simulink model "acvh_controller_mark0"  (R2020b)
settings: Solver=FixedStepAuto  StartTime=0.0  StopTime=Inf  RelTol=1e-3
values from neighbouring files (symbols this model uses):
  SampleTime = 0.001    [iris_quadcopter_specs.m]
undefined symbols (not defined in the file or in its folder): dev, Main, pwm_output0
libraries: pid_lib x6, px4uORBlib x5, sharedtransform x1, px4lib x1
settings Model: SimulationMode=external  EnablePacing=on  PacingRate=0.008900  ExtModeTrigDuration=10  Creator=sid  LastModifiedBy=sid
settings SolverCC: PositivePriorityOrder=on  AutoInsertRateTranBlk=on
settings OptimizationCC: EnhancedBackFolding=on  PassReuseOutputArgsAs=Individual arguments  ZeroExternalMemoryAtStartup=off  ZeroInternalMemoryAtStartup=off  MaxStackSize=64  OptimizeBlockOrder=speed  DifferentSizesBufferReuse=on  OptimizationCustomize=off  EfficientTunableParamExpr=on
settings DebuggingCC: ParameterTunabilityLossMsg=error
settings HardwareCC: ProdBitPerPointer=32  ProdBitPerSizeT=32  ProdBitPerPtrDiffT=32  ProdLargestAtomicInteger=Long  ProdLargestAtomicFloat=Double  ProdWordSize=32  ProdShiftRightIntArith=off  ProdLongLongMode=on  ProdHWDeviceType=ARM Compatible->ARM Cortex
settings SFSimCC: MATLABDynamicMemAlloc=off  SimTargetLang=C++
settings RTWCC: Description=Embedded Coder  SystemTargetFile=ert.tlc  HardwareBoard=PX4 Host Target  TLCOptions="-aInlineSetEventsForThisBaseRateFcn=TLC_FALSE -aSuppressMultiTaskScheduler=TLC_FALSE  -aRateBasedStepFcn=0"  TemplateMakefile=ert_default_tmf  Toolchain=GNU Tools for PX4 Autopilots  PortableWordSizes=on  TargetLang=C++
settings CodeAppCC: ForceParamTrailComments=on  IgnoreCustomStorageClasses=off  OperatorAnnotations=on  SimulinkDataObjDesc=on  SFDataObjDesc=on  InsertBlockDesc=on
settings ERTTargetCC: ExtMode=on  ExtModeMexArgs='127.0.0.1' 1 17725

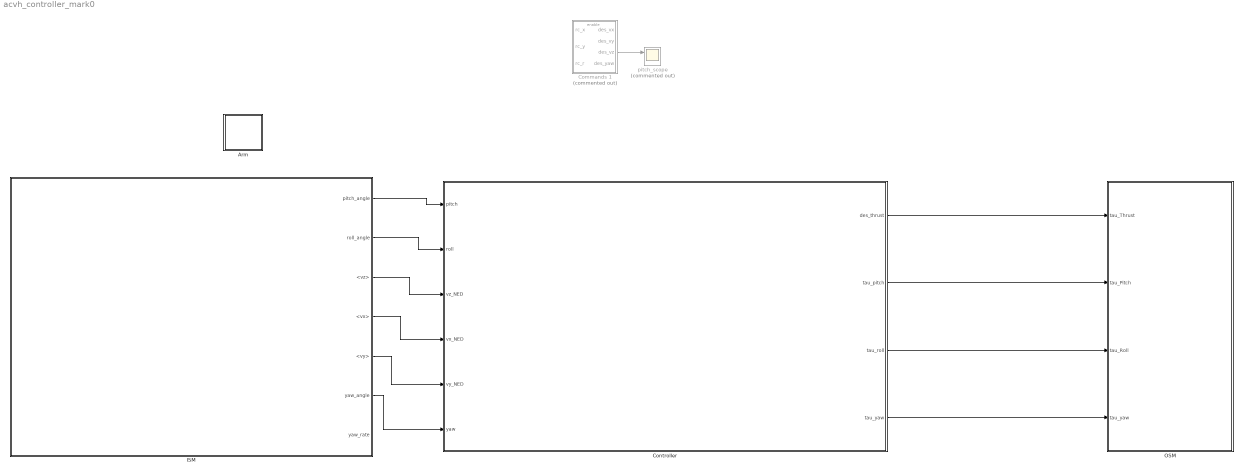
== system acvh_controller_mark0 ==
  Arm : Subsystem
  Commands 1 : Subsystem  Commented=on
  Controller : Subsystem
  ISM : Subsystem
  OSM : Subsystem
  pitch_scope : Scope  Commented=on  NumInputPorts=2
  wires:
  ISM/6(yaw_angle) -> Controller/6(yaw)
  ISM/1(pitch_angle) -> Controller/1(pitch)
  ISM/2(roll_angle) -> Controller/2(roll)
  ISM/3(<vz>) -> Controller/3(vz_NED)
  ISM/4(<vx>) -> Controller/4(vx_NED)
  ISM/5(<vy>) -> Controller/5(vy_NED)
  Controller/1(des_thrust) -> OSM/1(tau_Thrust)
  Controller/2(tau_pitch) -> OSM/2(tau_Pitch)
  Controller/3(tau_roll) -> OSM/3(tau_Roll)
  Controller/4(tau_yaw) -> OSM/4(tau_yaw)
  Commands 1/3(des_vz) -> pitch_scope/1

== system acvh_controller_mark0/Arm ==
  Bus Assignment : BusAssignment  AssignedSignals=armed
  Constant : Constant  OutDataTypeStr=Inherit: Inherit via back propagation  SampleTime=SampleTime
  Display1 : Display
  PX4 uORB Read : px4uORBlib/PX4 uORB Read  uORBTopic=actuator_armed  selectInstance=actuator_armed  SampleTime=SampleTime  BlockingMode=off  BlockTimeout=1e-3
      settings: SourceProductBaseCode=PX4AUTOPILOTS
  PX4 uORB Write : px4uORBlib/PX4 uORB Write  uORBTopic=actuator_armed  selectInstance=actuator_armed  MessageQueueLen=1
      settings: SourceProductBaseCode=PX4AUTOPILOTS
  wires:
  PX4 uORB Read/2 -> Bus Assignment/1
  PX4 uORB Read/1 -> Display1/1
  Bus Assignment/1 -> PX4 uORB Write/1
  Constant/1 -> Bus Assignment/2

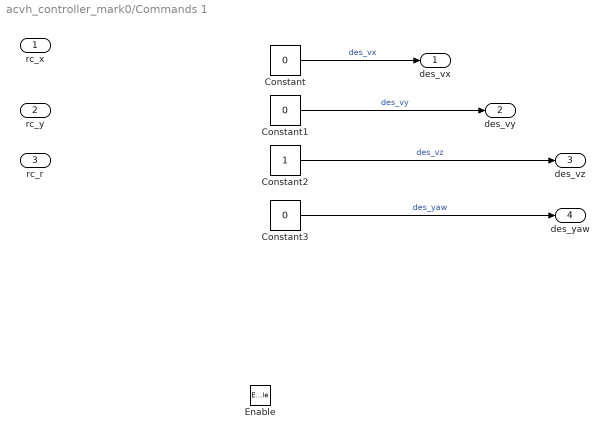
== system acvh_controller_mark0/Commands 1 ==
  rc_x : Inport
  rc_y : Inport  Port=2
  rc_r : Inport  Port=3
  Enable : EnablePort
  Constant : Constant  Value=0
  Constant1 : Constant  Value=0
  Constant2 : Constant
  Constant3 : Constant  Value=0
  des_vx : Outport
  des_vy : Outport  Port=2
  des_vz : Outport  Port=3
  des_yaw : Outport  Port=4
  wires:
  Constant1/1 -> des_vy/1  "des_vy"
  Constant/1 -> des_vx/1  "des_vx"
  Constant2/1 -> des_vz/1  "des_vz"
  Constant3/1 -> des_yaw/1  "des_yaw"

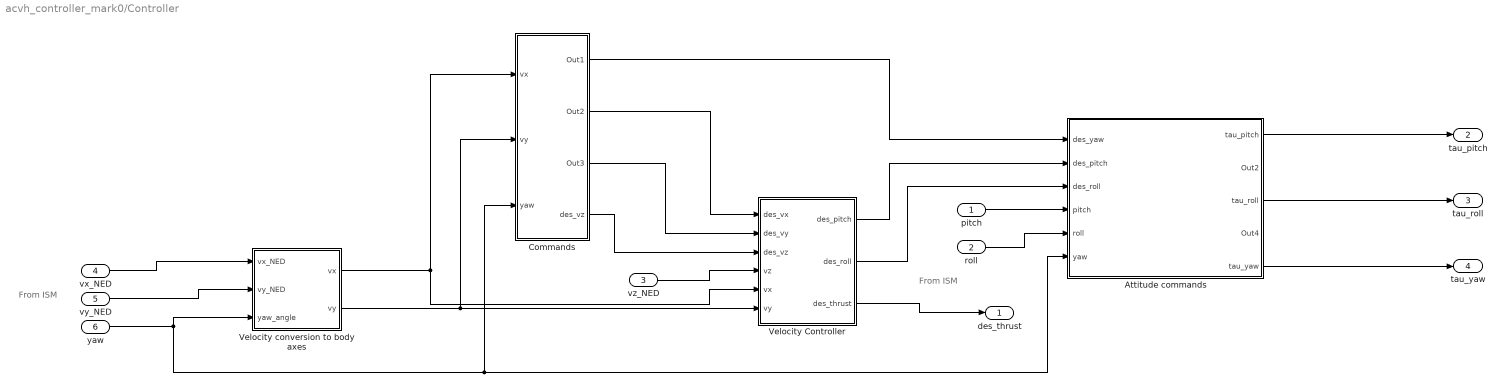
== system acvh_controller_mark0/Controller ==
  note: From ISM
  note: From ISM
  pitch : Inport
  roll : Inport  Port=2
  vz_NED : Inport  Port=3
  vx_NED : Inport  Port=4
  vy_NED : Inport  Port=5
  yaw : Inport  Port=6
  Attitude commands : Subsystem
  Commands : Subsystem
  Velocity Controller : Subsystem
  Velocity conversion to body axes : Subsystem
  des_thrust : Outport
  tau_pitch : Outport  Port=2
  tau_roll : Outport  Port=3
  tau_yaw : Outport  Port=4
  wires:
  vx_NED/1 -> Velocity conversion to body axes/1(vx_NED)
  pitch/1 -> Attitude commands/4(pitch)
  vy_NED/1 -> Velocity conversion to body axes/2(vy_NED)
  roll/1 -> Attitude commands/5(roll)
  yaw/1 -> Commands/3(yaw), Attitude commands/6(yaw), Velocity conversion to body axes/3(yaw_angle)
  vz_NED/1 -> Velocity Controller/4(vz)
  Velocity conversion to body axes/1(vx) -> Velocity Controller/5(vx), Commands/1(vx)
  Velocity conversion to body axes/2(vy) -> Commands/2(vy), Velocity Controller/6(vy)
  Attitude commands/1(tau_pitch) -> tau_pitch/1
  Attitude commands/3(tau_roll) -> tau_roll/1
  Attitude commands/5(tau_yaw) -> tau_yaw/1
  Velocity Controller/1(des_pitch) -> Attitude commands/2(des_pitch)
  Velocity Controller/2(des_roll) -> Attitude commands/3(des_roll)
  Velocity Controller/3(des_thrust) -> des_thrust/1
  Commands/1(Out1) -> Attitude commands/1(des_yaw)
  Commands/2(Out2) -> Velocity Controller/1(des_vx)
  Commands/3(Out3) -> Velocity Controller/2(des_vy)
  Commands/4(des_vz) -> Velocity Controller/3(des_vz)

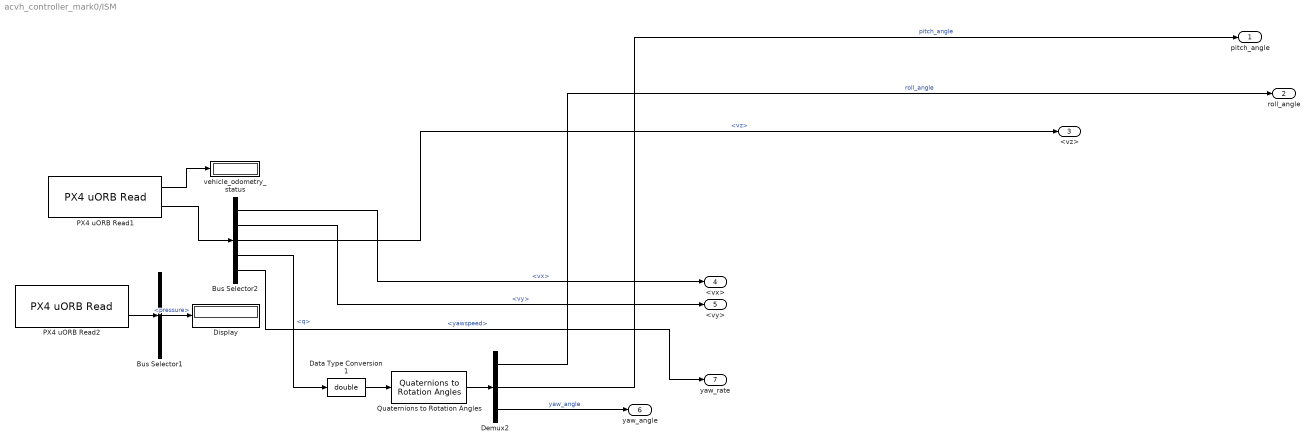
== system acvh_controller_mark0/ISM ==
  Bus Selector1 : BusSelector  OutputSignals=pressure
  Bus Selector2 : BusSelector  OutputSignals=vx,vy,vz,q,yawspeed
  Data Type Conversion1 : DataTypeConversion  OutDataTypeStr=double
  Demux2 : Demux  Outputs=3
  Display : Display
  PX4 uORB Read1 : px4uORBlib/PX4 uORB Read  uORBTopic=vehicle_odometry  selectInstance=vehicle_odometry  SampleTime=.001  BlockingMode=off  BlockTimeout=1e-3
      settings: SourceProductBaseCode=PX4AUTOPILOTS
  PX4 uORB Read2 : px4uORBlib/PX4 uORB Read  uORBTopic=sensor_baro  selectInstance=sensor_baro  SampleTime=.001  BlockingMode=off  BlockTimeout=1e-3
      settings: SourceProductBaseCode=PX4AUTOPILOTS
  Quaternions to Rotation Angles : sharedtransform/Quaternions to Rotation Angles  rotationOrder=XYZ  aMode=aMode
      settings: SourceProductBaseCode=AE,PW,MT,UV,VE,VP
  vehicle_odometry_status : Display
  pitch_angle : Outport
  roll_angle : Outport  Port=2
  <vz> : Outport  Port=3
  <vx> : Outport  Port=4
  <vy> : Outport  Port=5
  yaw_angle : Outport  Port=6
  yaw_rate : Outport  Port=7
  wires:
  PX4 uORB Read1/1 -> vehicle_odometry_status/1
  Bus Selector2/4 -> Data Type Conversion1/1  "<q>"
  PX4 uORB Read1/2 -> Bus Selector2/1
  Bus Selector2/2 -> <vy>/1  "<vy>"
  Bus Selector2/3 -> <vz>/1  "<vz>"
  Demux2/2 -> pitch_angle/1  "pitch_angle"
  Bus Selector2/1 -> <vx>/1  "<vx>"
  Demux2/3 -> yaw_angle/1  "yaw_angle"
  Data Type Conversion1/1 -> Quaternions to Rotation Angles/1
  Quaternions to Rotation Angles/1 -> Demux2/1
  Demux2/1 -> roll_angle/1  "roll_angle"
  PX4 uORB Read2/2 -> Bus Selector1/1
  Bus Selector1/1 -> Display/1  "<pressure>"
  Bus Selector2/5 -> yaw_rate/1  "<yawspeed>"

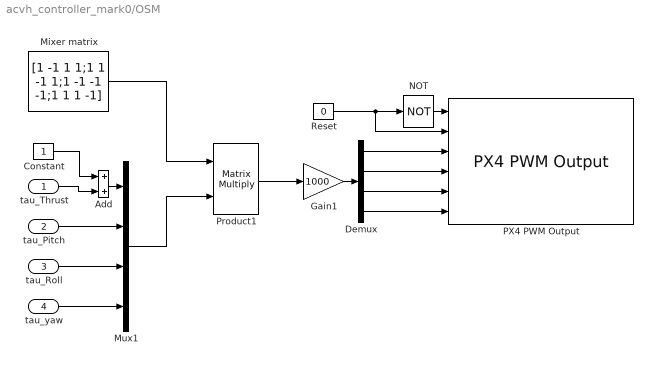
== system acvh_controller_mark0/OSM ==
  tau_Thrust : Inport
  tau_Pitch : Inport  Port=2
  tau_Roll : Inport  Port=3
  tau_yaw : Inport  Port=4
  Add : Sum
  Constant : Constant
  Demux : Demux
  Gain1 : Gain  Gain=1000  OutDataTypeStr=uint16
  Mixer matrix : Constant  Value=[1 -1 1 1;1 1 -1 1;1 -1 -1 -1;1 1 1 -1]  OutDataTypeStr=Inherit: Inherit via back propagation
  Mux1 : Mux
  NOT : Logic  Operator=NOT  IconShape=distinctive  AllPortsSameDT=off  OutDataTypeStr=boolean
  PX4 PWM Output : px4lib/PX4 PWM Output  pwmDevice=Main (/dev/pwm_output0)  pwmChannel1_=on  pwmChannel2_=on  pwmChannel3_=on  pwmChannel4_=on  pwmChannel5_=off  pwmChannel6_=off  pwmChannel7_=off  pwmChannel8_=off  forceTerminateFailsafe=off  outputErrorStatus=off
      settings: SourceProductBaseCode=PX4AUTOPILOTS
  Product1 : Product  Multiplication=Matrix(*)  RndMeth=Zero
  Reset : Constant  Value=0  OutDataTypeStr=boolean
  wires:
  NOT/1 -> PX4 PWM Output/1
  Mixer matrix/1 -> Product1/1
  tau_yaw/1 -> Mux1/4
  tau_Pitch/1 -> Mux1/2
  tau_Roll/1 -> Mux1/3
  Reset/1 -> PX4 PWM Output/2, NOT/1
  Demux/3 -> PX4 PWM Output/5
  Demux/2 -> PX4 PWM Output/4
  Mux1/1 -> Product1/2
  Demux/4 -> PX4 PWM Output/6
  Gain1/1 -> Demux/1
  Demux/1 -> PX4 PWM Output/3
  Product1/1 -> Gain1/1
  tau_Thrust/1 -> Add/2
  Add/1 -> Mux1/1
  Constant/1 -> Add/1

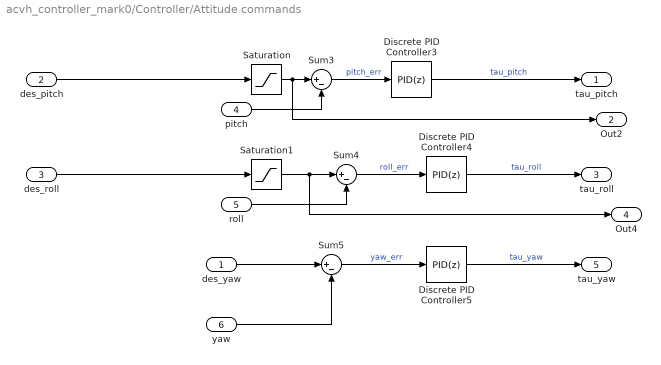
== system acvh_controller_mark0/Controller/Attitude commands ==
  des_yaw : Inport
  des_pitch : Inport  Port=2
  des_roll : Inport  Port=3
  pitch : Inport  Port=4
  roll : Inport  Port=5
  yaw : Inport  Port=6
  Discrete PID Controller3 : pid_lib/PID Controller  Controller=PID  Form=Parallel  TimeDomain=Discrete-time  UseExternalTs=off  SampleTime=-1  IntegratorMethod=Forward Euler  FilterMethod=Forward Euler  ControllerParametersSource=internal  P=1  I=1  D=0  UseFilter=on  N=100  TunerSelectOption=Transfer Function Based (PID Tuner App)  InitialConditionSource=internal  InitialConditionForIntegrator=0  InitialConditionForFilter=0  DifferentiatorICPrevScaledInput=0  ExternalReset=none  TrackingMode=off  Kt=1  LimitOutput=on  SatLimitsSource=internal  UpperSaturationLimit=.05  LowerSaturationLimit=-.05  LinearizeAsGain=off  AntiWindupMode=none  Kb=1  POutMin=[]  POutMax=[]  IOutMin=[]  IOutMax=[]  DOutMin=[]  DOutMax=[]  NOutMin=[]  NOutMax=[]  SumOutMin=[]  SumOutMax=[]  SaturationOutMin=[]  SaturationOutMax=[]  PParamMin=[]  PParamMax=[]  IParamMin=[]  IParamMax=[]  DParamMin=[]  DParamMax=[]  NParamMin=[]  NParamMax=[]  KbParamMin=[]  KbParamMax=[]  KtParamMin=[]  KtParamMax=[]  KbOutMin=[]  KbOutMax=[]  KtOutMin=[]  KtOutMax=[]  IntegratorOutMin=[]  IntegratorOutMax=[]  FilterOutMin=[]  FilterOutMax=[]  SumI1OutMin=[]  SumI1OutMax=[]  SumI2OutMin=[]  SumI2OutMax=[]  SumI3OutMin=[]  SumI3OutMax=[]  SumI4OutMin=[]  SumI4OutMax=[]  SumDOutMin=[]  SumDOutMax=[]  DifferentiatorOutMin=[]  DifferentiatorOutMax=[]  FilterDiffOutCoefMin=[]  FilterDiffOutCoefMax=[]  ReciprocalOutMin=[]  ReciprocalOutMax=[]  SumDenOutMin=[]  SumDenOutMax=[]  SumNumOutMin=[]  SumNumOutMax=[]  DivideOutMin=[]  DivideOutMax=[]  UdiffTsProdOutMin=[]  UdiffTsProdOutMax=[]  NTsProdOutMin=[]  NTsProdOutMax=[]  UintegralTsProdOutMin=[]  UintegralTsProdOutMax=[]  UngainTsProdOutMin=[]  UngainTsProdOutMax=[]  IntegratorContinuousStateAttributes=''  IntegratorStateMustResolveToSignalObject=off  IntegratorRTWStateStorageClass=Auto  FilterContinuousStateAttributes=''  FilterStateMustResolveToSignalObject=off  FilterRTWStateStorageClass=Auto  ParallelPVariant=InternalParameters  IdealPVariant=Disabled  IVariant=InternalParameters  DVariant=InternalParameters  IntegratorVariant=Discrete  SatVariant=Enabled  AWVariant=Passthrough  PCopyVariant=Disabled  TRVariant=Disabled  FdbkBlocksVariant=Forward  IdealPFdbkVariant=Disabled  SatFdbkVariant=Disabled  DerivativeFilterVariant=ForwardEulerFilter  NVariant=InternalParameters  NCopyVariant=Disabled  FilterICVariant=InternalICsFilter  IntegratorICVariant=InternalICs  ExternalResetVariant=Disabled  TRSumVariant=Passthrough  SumFdbkVariant=Disabled  SumVariant=Sum_PID  TsampFilterVariant=InternalTs  TsampNgainVariant=Passthrough  TsampIntegralVariant=Passthrough  ExternalSaturationOutDataTypeStr=Inherit: Same as second input
  Discrete PID Controller4 : pid_lib/PID Controller  Controller=PID  Form=Parallel  TimeDomain=Discrete-time  UseExternalTs=off  SampleTime=-1  IntegratorMethod=Forward Euler  FilterMethod=Forward Euler  ControllerParametersSource=internal  P=1  I=1  D=0  UseFilter=on  N=100  TunerSelectOption=Transfer Function Based (PID Tuner App)  InitialConditionSource=internal  InitialConditionForIntegrator=0  InitialConditionForFilter=0  DifferentiatorICPrevScaledInput=0  ExternalReset=none  TrackingMode=off  Kt=1  LimitOutput=on  SatLimitsSource=internal  UpperSaturationLimit=.05  LowerSaturationLimit=-.05  LinearizeAsGain=off  AntiWindupMode=none  Kb=1  POutMin=[]  POutMax=[]  IOutMin=[]  IOutMax=[]  DOutMin=[]  DOutMax=[]  NOutMin=[]  NOutMax=[]  SumOutMin=[]  SumOutMax=[]  SaturationOutMin=[]  SaturationOutMax=[]  PParamMin=[]  PParamMax=[]  IParamMin=[]  IParamMax=[]  DParamMin=[]  DParamMax=[]  NParamMin=[]  NParamMax=[]  KbParamMin=[]  KbParamMax=[]  KtParamMin=[]  KtParamMax=[]  KbOutMin=[]  KbOutMax=[]  KtOutMin=[]  KtOutMax=[]  IntegratorOutMin=[]  IntegratorOutMax=[]  FilterOutMin=[]  FilterOutMax=[]  SumI1OutMin=[]  SumI1OutMax=[]  SumI2OutMin=[]  SumI2OutMax=[]  SumI3OutMin=[]  SumI3OutMax=[]  SumI4OutMin=[]  SumI4OutMax=[]  SumDOutMin=[]  SumDOutMax=[]  DifferentiatorOutMin=[]  DifferentiatorOutMax=[]  FilterDiffOutCoefMin=[]  FilterDiffOutCoefMax=[]  ReciprocalOutMin=[]  ReciprocalOutMax=[]  SumDenOutMin=[]  SumDenOutMax=[]  SumNumOutMin=[]  SumNumOutMax=[]  DivideOutMin=[]  DivideOutMax=[]  UdiffTsProdOutMin=[]  UdiffTsProdOutMax=[]  NTsProdOutMin=[]  NTsProdOutMax=[]  UintegralTsProdOutMin=[]  UintegralTsProdOutMax=[]  UngainTsProdOutMin=[]  UngainTsProdOutMax=[]  IntegratorContinuousStateAttributes=''  IntegratorStateMustResolveToSignalObject=off  IntegratorRTWStateStorageClass=Auto  FilterContinuousStateAttributes=''  FilterStateMustResolveToSignalObject=off  FilterRTWStateStorageClass=Auto  ParallelPVariant=InternalParameters  IdealPVariant=Disabled  IVariant=InternalParameters  DVariant=InternalParameters  IntegratorVariant=Discrete  SatVariant=Enabled  AWVariant=Passthrough  PCopyVariant=Disabled  TRVariant=Disabled  FdbkBlocksVariant=Forward  IdealPFdbkVariant=Disabled  SatFdbkVariant=Disabled  DerivativeFilterVariant=ForwardEulerFilter  NVariant=InternalParameters  NCopyVariant=Disabled  FilterICVariant=InternalICsFilter  IntegratorICVariant=InternalICs  ExternalResetVariant=Disabled  TRSumVariant=Passthrough  SumFdbkVariant=Disabled  SumVariant=Sum_PID  TsampFilterVariant=InternalTs  TsampNgainVariant=Passthrough  TsampIntegralVariant=Passthrough  ExternalSaturationOutDataTypeStr=Inherit: Same as second input
  Discrete PID Controller5 : pid_lib/PID Controller  Controller=PID  Form=Parallel  TimeDomain=Discrete-time  UseExternalTs=off  SampleTime=-1  IntegratorMethod=Forward Euler  FilterMethod=Forward Euler  ControllerParametersSource=internal  P=1  I=1  D=0  UseFilter=on  N=100  TunerSelectOption=Transfer Function Based (PID Tuner App)  InitialConditionSource=internal  InitialConditionForIntegrator=0  InitialConditionForFilter=0  DifferentiatorICPrevScaledInput=0  ExternalReset=none  TrackingMode=off  Kt=1  LimitOutput=on  SatLimitsSource=internal  UpperSaturationLimit=0.1  LowerSaturationLimit=-0.1  LinearizeAsGain=off  AntiWindupMode=none  Kb=1  POutMin=[]  POutMax=[]  IOutMin=[]  IOutMax=[]  DOutMin=[]  DOutMax=[]  NOutMin=[]  NOutMax=[]  SumOutMin=[]  SumOutMax=[]  SaturationOutMin=[]  SaturationOutMax=[]  PParamMin=[]  PParamMax=[]  IParamMin=[]  IParamMax=[]  DParamMin=[]  DParamMax=[]  NParamMin=[]  NParamMax=[]  KbParamMin=[]  KbParamMax=[]  KtParamMin=[]  KtParamMax=[]  KbOutMin=[]  KbOutMax=[]  KtOutMin=[]  KtOutMax=[]  IntegratorOutMin=[]  IntegratorOutMax=[]  FilterOutMin=[]  FilterOutMax=[]  SumI1OutMin=[]  SumI1OutMax=[]  SumI2OutMin=[]  SumI2OutMax=[]  SumI3OutMin=[]  SumI3OutMax=[]  SumI4OutMin=[]  SumI4OutMax=[]  SumDOutMin=[]  SumDOutMax=[]  DifferentiatorOutMin=[]  DifferentiatorOutMax=[]  FilterDiffOutCoefMin=[]  FilterDiffOutCoefMax=[]  ReciprocalOutMin=[]  ReciprocalOutMax=[]  SumDenOutMin=[]  SumDenOutMax=[]  SumNumOutMin=[]  SumNumOutMax=[]  DivideOutMin=[]  DivideOutMax=[]  UdiffTsProdOutMin=[]  UdiffTsProdOutMax=[]  NTsProdOutMin=[]  NTsProdOutMax=[]  UintegralTsProdOutMin=[]  UintegralTsProdOutMax=[]  UngainTsProdOutMin=[]  UngainTsProdOutMax=[]  IntegratorContinuousStateAttributes=''  IntegratorStateMustResolveToSignalObject=off  IntegratorRTWStateStorageClass=Auto  FilterContinuousStateAttributes=''  FilterStateMustResolveToSignalObject=off  FilterRTWStateStorageClass=Auto  ParallelPVariant=InternalParameters  IdealPVariant=Disabled  IVariant=InternalParameters  DVariant=InternalParameters  IntegratorVariant=Discrete  SatVariant=Enabled  AWVariant=Passthrough  PCopyVariant=Disabled  TRVariant=Disabled  FdbkBlocksVariant=Forward  IdealPFdbkVariant=Disabled  SatFdbkVariant=Disabled  DerivativeFilterVariant=ForwardEulerFilter  NVariant=InternalParameters  NCopyVariant=Disabled  FilterICVariant=InternalICsFilter  IntegratorICVariant=InternalICs  ExternalResetVariant=Disabled  TRSumVariant=Passthrough  SumFdbkVariant=Disabled  SumVariant=Sum_PID  TsampFilterVariant=InternalTs  TsampNgainVariant=Passthrough  TsampIntegralVariant=Passthrough  ExternalSaturationOutDataTypeStr=Inherit: Same as second input
  Saturation : Saturate  UpperLimit=pi/4  LowerLimit=-pi/4
  Saturation1 : Saturate  UpperLimit=pi/4  LowerLimit=-pi/4
  Sum3 : Sum  Inputs=|+-
  Sum4 : Sum  Inputs=|+-
  Sum5 : Sum  Inputs=|+-
  tau_pitch : Outport
  Out2 : Outport  Port=2
  tau_roll : Outport  Port=3
  Out4 : Outport  Port=4
  tau_yaw : Outport  Port=5
  wires:
  Discrete PID Controller5/1 -> tau_yaw/1  "tau_yaw"
  roll/1 -> Sum4/2
  yaw/1 -> Sum5/2
  des_roll/1 -> Saturation1/1
  des_yaw/1 -> Sum5/1
  Discrete PID Controller4/1 -> tau_roll/1  "tau_roll"
  Sum5/1 -> Discrete PID Controller5/1  "yaw_err"
  Sum4/1 -> Discrete PID Controller4/1  "roll_err"
  des_pitch/1 -> Saturation/1
  pitch/1 -> Sum3/2
  Saturation1/1 -> Out4/1, Sum4/1
  Saturation/1 -> Out2/1, Sum3/1
  Discrete PID Controller3/1 -> tau_pitch/1  "tau_pitch"
  Sum3/1 -> Discrete PID Controller3/1  "pitch_err"

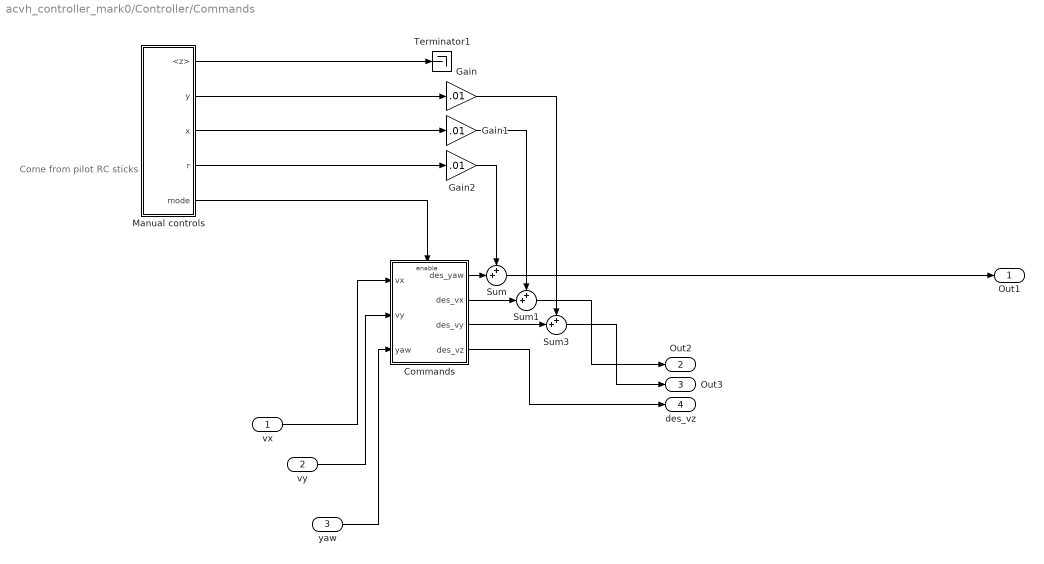
== system acvh_controller_mark0/Controller/Commands ==
  note: Come from pilot RC sticks
  vx : Inport
  vy : Inport  Port=2
  yaw : Inport  Port=3
  "Commands " : Subsystem
  Gain : Gain  Gain=.01
  Gain1 : Gain  Gain=.01
  Gain2 : Gain  Gain=.01
  Manual controls : Subsystem
  Sum : Sum  Inputs=++|
  Sum1 : Sum  Inputs=++|
  Sum3 : Sum  Inputs=++|
  Terminator1 : Terminator
  Out1 : Outport
  Out2 : Outport  Port=2
  Out3 : Outport  Port=3
  des_vz : Outport  Port=4
  wires:
  Gain/1 -> Sum3/1
  "Commands "/4(des_vz) -> des_vz/1
  Manual controls/4(r) -> Gain2/1
  "Commands "/2(des_vx) -> Sum1/2
  Manual controls/5(mode) -> "Commands "/Enable
  Sum3/1 -> Out3/1
  "Commands "/1(des_yaw) -> Sum/2
  Manual controls/1(<z>) -> Terminator1/1
  Sum1/1 -> Out2/1
  Gain2/1 -> Sum/1
  Sum/1 -> Out1/1
  yaw/1 -> "Commands "/3(yaw)
  vy/1 -> "Commands "/2(vy)
  Manual controls/2(y) -> Gain/1
  "Commands "/3(des_vy) -> Sum3/2
  vx/1 -> "Commands "/1(vx)
  Manual controls/3(x) -> Gain1/1
  Gain1/1 -> Sum1/1

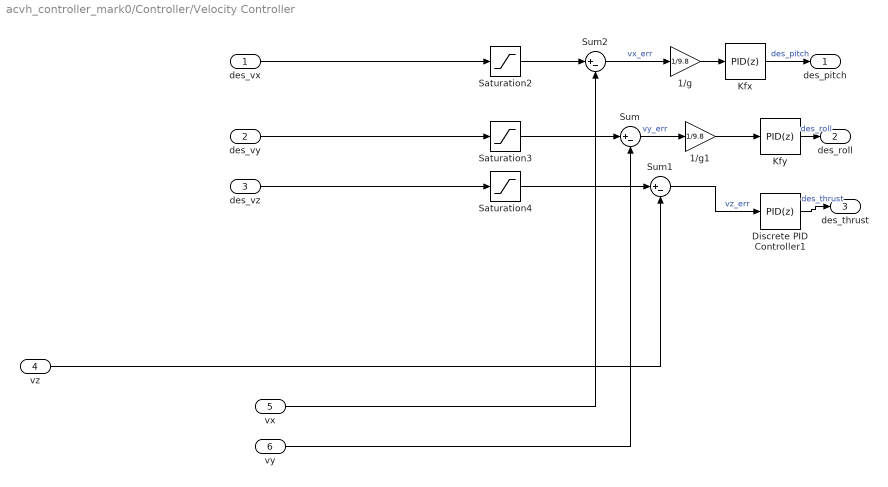
== system acvh_controller_mark0/Controller/Velocity Controller ==
  des_vx : Inport
  des_vy : Inport  Port=2
  des_vz : Inport  Port=3
  vz : Inport  Port=4
  vx : Inport  Port=5
  vy : Inport  Port=6
  1/g : Gain  Gain=1/9.8
  1/g1 : Gain  Gain=1/9.8
  Discrete PID Controller1 : pid_lib/PID Controller  Controller=PID  Form=Parallel  TimeDomain=Discrete-time  UseExternalTs=off  SampleTime=-1  IntegratorMethod=Forward Euler  FilterMethod=Forward Euler  ControllerParametersSource=internal  P=4  I=2  D=0  UseFilter=on  N=100  TunerSelectOption=Transfer Function Based (PID Tuner App)  InitialConditionSource=internal  InitialConditionForIntegrator=0  InitialConditionForFilter=0  DifferentiatorICPrevScaledInput=0  ExternalReset=none  TrackingMode=off  Kt=1  LimitOutput=off  SatLimitsSource=internal  UpperSaturationLimit=inf  LowerSaturationLimit=-inf  LinearizeAsGain=off  AntiWindupMode=none  Kb=1  POutMin=[]  POutMax=[]  IOutMin=[]  IOutMax=[]  DOutMin=[]  DOutMax=[]  NOutMin=[]  NOutMax=[]  SumOutMin=[]  SumOutMax=[]  SaturationOutMin=[]  SaturationOutMax=[]  PParamMin=[]  PParamMax=[]  IParamMin=[]  IParamMax=[]  DParamMin=[]  DParamMax=[]  NParamMin=[]  NParamMax=[]  KbParamMin=[]  KbParamMax=[]  KtParamMin=[]  KtParamMax=[]  KbOutMin=[]  KbOutMax=[]  KtOutMin=[]  KtOutMax=[]  IntegratorOutMin=[]  IntegratorOutMax=[]  FilterOutMin=[]  FilterOutMax=[]  SumI1OutMin=[]  SumI1OutMax=[]  SumI2OutMin=[]  SumI2OutMax=[]  SumI3OutMin=[]  SumI3OutMax=[]  SumI4OutMin=[]  SumI4OutMax=[]  SumDOutMin=[]  SumDOutMax=[]  DifferentiatorOutMin=[]  DifferentiatorOutMax=[]  FilterDiffOutCoefMin=[]  FilterDiffOutCoefMax=[]  ReciprocalOutMin=[]  ReciprocalOutMax=[]  SumDenOutMin=[]  SumDenOutMax=[]  SumNumOutMin=[]  SumNumOutMax=[]  DivideOutMin=[]  DivideOutMax=[]  UdiffTsProdOutMin=[]  UdiffTsProdOutMax=[]  NTsProdOutMin=[]  NTsProdOutMax=[]  UintegralTsProdOutMin=[]  UintegralTsProdOutMax=[]  UngainTsProdOutMin=[]  UngainTsProdOutMax=[]  IntegratorContinuousStateAttributes=''  IntegratorStateMustResolveToSignalObject=off  IntegratorRTWStateStorageClass=Auto  FilterContinuousStateAttributes=''  FilterStateMustResolveToSignalObject=off  FilterRTWStateStorageClass=Auto  ParallelPVariant=InternalParameters  IdealPVariant=Disabled  IVariant=InternalParameters  DVariant=InternalParameters  IntegratorVariant=Discrete  SatVariant=Disabled  AWVariant=Passthrough  PCopyVariant=Disabled  TRVariant=Disabled  FdbkBlocksVariant=Forward  IdealPFdbkVariant=Disabled  SatFdbkVariant=Disabled  DerivativeFilterVariant=ForwardEulerFilter  NVariant=InternalParameters  NCopyVariant=Disabled  FilterICVariant=InternalICsFilter  IntegratorICVariant=InternalICs  ExternalResetVariant=Disabled  TRSumVariant=Passthrough  SumFdbkVariant=Disabled  SumVariant=Sum_PID  TsampFilterVariant=InternalTs  TsampNgainVariant=Passthrough  TsampIntegralVariant=Passthrough  ExternalSaturationOutDataTypeStr=Inherit: Same as second input
  Kfx : pid_lib/PID Controller  Controller=PID  Form=Parallel  TimeDomain=Discrete-time  UseExternalTs=off  SampleTime=-1  IntegratorMethod=Forward Euler  FilterMethod=Forward Euler  ControllerParametersSource=internal  P=1.8  I=0  D=0  UseFilter=on  N=100  TunerSelectOption=Transfer Function Based (PID Tuner App)  InitialConditionSource=internal  InitialConditionForIntegrator=0  InitialConditionForFilter=0  DifferentiatorICPrevScaledInput=0  ExternalReset=none  TrackingMode=off  Kt=1  LimitOutput=off  SatLimitsSource=internal  UpperSaturationLimit=inf  LowerSaturationLimit=-inf  LinearizeAsGain=off  AntiWindupMode=none  Kb=1  POutMin=[]  POutMax=[]  IOutMin=[]  IOutMax=[]  DOutMin=[]  DOutMax=[]  NOutMin=[]  NOutMax=[]  SumOutMin=[]  SumOutMax=[]  SaturationOutMin=[]  SaturationOutMax=[]  PParamMin=[]  PParamMax=[]  IParamMin=[]  IParamMax=[]  DParamMin=[]  DParamMax=[]  NParamMin=[]  NParamMax=[]  KbParamMin=[]  KbParamMax=[]  KtParamMin=[]  KtParamMax=[]  KbOutMin=[]  KbOutMax=[]  KtOutMin=[]  KtOutMax=[]  IntegratorOutMin=[]  IntegratorOutMax=[]  FilterOutMin=[]  FilterOutMax=[]  SumI1OutMin=[]  SumI1OutMax=[]  SumI2OutMin=[]  SumI2OutMax=[]  SumI3OutMin=[]  SumI3OutMax=[]  SumI4OutMin=[]  SumI4OutMax=[]  SumDOutMin=[]  SumDOutMax=[]  DifferentiatorOutMin=[]  DifferentiatorOutMax=[]  FilterDiffOutCoefMin=[]  FilterDiffOutCoefMax=[]  ReciprocalOutMin=[]  ReciprocalOutMax=[]  SumDenOutMin=[]  SumDenOutMax=[]  SumNumOutMin=[]  SumNumOutMax=[]  DivideOutMin=[]  DivideOutMax=[]  UdiffTsProdOutMin=[]  UdiffTsProdOutMax=[]  NTsProdOutMin=[]  NTsProdOutMax=[]  UintegralTsProdOutMin=[]  UintegralTsProdOutMax=[]  UngainTsProdOutMin=[]  UngainTsProdOutMax=[]  IntegratorContinuousStateAttributes=''  IntegratorStateMustResolveToSignalObject=off  IntegratorRTWStateStorageClass=Auto  FilterContinuousStateAttributes=''  FilterStateMustResolveToSignalObject=off  FilterRTWStateStorageClass=Auto  ParallelPVariant=InternalParameters  IdealPVariant=Disabled  IVariant=InternalParameters  DVariant=InternalParameters  IntegratorVariant=Discrete  SatVariant=Disabled  AWVariant=Passthrough  PCopyVariant=Disabled  TRVariant=Disabled  FdbkBlocksVariant=Forward  IdealPFdbkVariant=Disabled  SatFdbkVariant=Disabled  DerivativeFilterVariant=ForwardEulerFilter  NVariant=InternalParameters  NCopyVariant=Disabled  FilterICVariant=InternalICsFilter  IntegratorICVariant=InternalICs  ExternalResetVariant=Disabled  TRSumVariant=Passthrough  SumFdbkVariant=Disabled  SumVariant=Sum_PID  TsampFilterVariant=InternalTs  TsampNgainVariant=Passthrough  TsampIntegralVariant=Passthrough  ExternalSaturationOutDataTypeStr=Inherit: Same as second input
  Kfy : pid_lib/PID Controller  Controller=PID  Form=Parallel  TimeDomain=Discrete-time  UseExternalTs=off  SampleTime=-1  IntegratorMethod=Forward Euler  FilterMethod=Forward Euler  ControllerParametersSource=internal  P=1.8  I=0  D=0  UseFilter=on  N=100  TunerSelectOption=Transfer Function Based (PID Tuner App)  InitialConditionSource=internal  InitialConditionForIntegrator=0  InitialConditionForFilter=0  DifferentiatorICPrevScaledInput=0  ExternalReset=none  TrackingMode=off  Kt=1  LimitOutput=off  SatLimitsSource=internal  UpperSaturationLimit=inf  LowerSaturationLimit=-inf  LinearizeAsGain=off  AntiWindupMode=none  Kb=1  POutMin=[]  POutMax=[]  IOutMin=[]  IOutMax=[]  DOutMin=[]  DOutMax=[]  NOutMin=[]  NOutMax=[]  SumOutMin=[]  SumOutMax=[]  SaturationOutMin=[]  SaturationOutMax=[]  PParamMin=[]  PParamMax=[]  IParamMin=[]  IParamMax=[]  DParamMin=[]  DParamMax=[]  NParamMin=[]  NParamMax=[]  KbParamMin=[]  KbParamMax=[]  KtParamMin=[]  KtParamMax=[]  KbOutMin=[]  KbOutMax=[]  KtOutMin=[]  KtOutMax=[]  IntegratorOutMin=[]  IntegratorOutMax=[]  FilterOutMin=[]  FilterOutMax=[]  SumI1OutMin=[]  SumI1OutMax=[]  SumI2OutMin=[]  SumI2OutMax=[]  SumI3OutMin=[]  SumI3OutMax=[]  SumI4OutMin=[]  SumI4OutMax=[]  SumDOutMin=[]  SumDOutMax=[]  DifferentiatorOutMin=[]  DifferentiatorOutMax=[]  FilterDiffOutCoefMin=[]  FilterDiffOutCoefMax=[]  ReciprocalOutMin=[]  ReciprocalOutMax=[]  SumDenOutMin=[]  SumDenOutMax=[]  SumNumOutMin=[]  SumNumOutMax=[]  DivideOutMin=[]  DivideOutMax=[]  UdiffTsProdOutMin=[]  UdiffTsProdOutMax=[]  NTsProdOutMin=[]  NTsProdOutMax=[]  UintegralTsProdOutMin=[]  UintegralTsProdOutMax=[]  UngainTsProdOutMin=[]  UngainTsProdOutMax=[]  IntegratorContinuousStateAttributes=''  IntegratorStateMustResolveToSignalObject=off  IntegratorRTWStateStorageClass=Auto  FilterContinuousStateAttributes=''  FilterStateMustResolveToSignalObject=off  FilterRTWStateStorageClass=Auto  ParallelPVariant=InternalParameters  IdealPVariant=Disabled  IVariant=InternalParameters  DVariant=InternalParameters  IntegratorVariant=Discrete  SatVariant=Disabled  AWVariant=Passthrough  PCopyVariant=Disabled  TRVariant=Disabled  FdbkBlocksVariant=Forward  IdealPFdbkVariant=Disabled  SatFdbkVariant=Disabled  DerivativeFilterVariant=ForwardEulerFilter  NVariant=InternalParameters  NCopyVariant=Disabled  FilterICVariant=InternalICsFilter  IntegratorICVariant=InternalICs  ExternalResetVariant=Disabled  TRSumVariant=Passthrough  SumFdbkVariant=Disabled  SumVariant=Sum_PID  TsampFilterVariant=InternalTs  TsampNgainVariant=Passthrough  TsampIntegralVariant=Passthrough  ExternalSaturationOutDataTypeStr=Inherit: Same as second input
  Saturation2 : Saturate  UpperLimit=12  LowerLimit=-12
  Saturation3 : Saturate  UpperLimit=12  LowerLimit=-12
  Saturation4 : Saturate  UpperLimit=1  LowerLimit=-3
  Sum : Sum  Inputs=|+-
  Sum1 : Sum  Inputs=|+-
  Sum2 : Sum  Inputs=|+-
  des_pitch : Outport
  des_roll : Outport  Port=2
  des_thrust : Outport  Port=3
  wires:
  Sum2/1 -> 1/g/1  "vx_err"
  Sum1/1 -> Discrete PID Controller1/1  "vz_err"
  Saturation4/1 -> Sum1/1
  Kfy/1 -> des_roll/1  "des_roll"
  Saturation3/1 -> Sum/1
  Sum/1 -> 1/g1/1  "vy_err"
  vx/1 -> Sum2/2
  des_vx/1 -> Saturation2/1
  Saturation2/1 -> Sum2/1
  des_vy/1 -> Saturation3/1
  Kfx/1 -> des_pitch/1  "des_pitch"
  vy/1 -> Sum/2
  vz/1 -> Sum1/2
  des_vz/1 -> Saturation4/1
  Discrete PID Controller1/1 -> des_thrust/1  "des_thrust"
  1/g/1 -> Kfx/1
  1/g1/1 -> Kfy/1

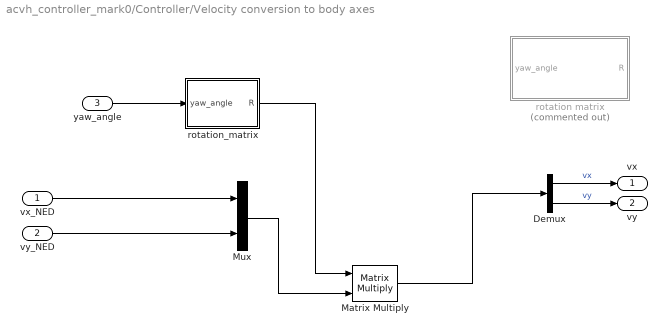
== system acvh_controller_mark0/Controller/Velocity conversion to body axes ==
  vx_NED : Inport
  vy_NED : Inport  Port=2
  yaw_angle : Inport  Port=3
  Demux : Demux  Outputs=2
  Matrix Multiply : Product  Multiplication=Matrix(*)
  Mux : Mux  Inputs=2
  rotation matrix : Subsystem  Commented=on
  rotation_matrix : MATLAB Function  TreatAsAtomicUnit=on  SystemSampleTime=SampleTime
  vx : Outport
  vy : Outport  Port=2
  wires:
  vy_NED/1 -> Mux/2
  vx_NED/1 -> Mux/1
  Demux/1 -> vx/1  "vx"
  Demux/2 -> vy/1  "vy"
  rotation_matrix/1(R) -> Matrix Multiply/1
  Matrix Multiply/1 -> Demux/1
  yaw_angle/1 -> rotation_matrix/1(yaw_angle)
  Mux/1 -> Matrix Multiply/2

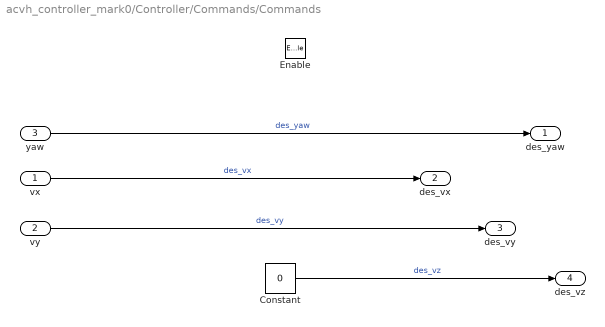
== system acvh_controller_mark0/Controller/Commands/Commands  ==
  vx : Inport
  vy : Inport  Port=2
  yaw : Inport  Port=3
  Enable : EnablePort
  Constant : Constant  Value=0
  des_yaw : Outport
  des_vx : Outport  Port=2
  des_vy : Outport  Port=3
  des_vz : Outport  Port=4
  wires:
  vy/1 -> des_vy/1  "des_vy"
  vx/1 -> des_vx/1  "des_vx"
  Constant/1 -> des_vz/1  "des_vz"
  yaw/1 -> des_yaw/1  "des_yaw"

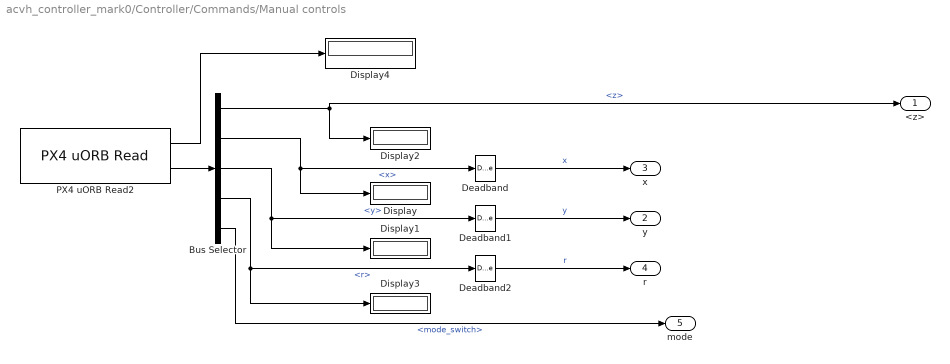
== system acvh_controller_mark0/Controller/Commands/Manual controls ==
  Bus Selector : BusSelector  OutputSignals=z,x,y,r,mode_switch
  Deadband : DeadZone  LowerValue=-0.05  UpperValue=0.05  SaturateOnIntegerOverflow=on
  Deadband1 : DeadZone  LowerValue=-0.05  UpperValue=0.05  SaturateOnIntegerOverflow=on
  Deadband2 : DeadZone  LowerValue=-0.05  UpperValue=0.05  SaturateOnIntegerOverflow=on
  Display{,1..4} (5 alike) : Display
  PX4 uORB Read2 : px4uORBlib/PX4 uORB Read  uORBTopic=manual_control_setpoint  selectInstance=manual_control_setpoint  SampleTime=SampleTime  BlockingMode=off  BlockTimeout=1e-3
      settings: SourceProductBaseCode=PX4AUTOPILOTS
  <z> : Outport
  y : Outport  Port=2
  x : Outport  Port=3
  r : Outport  Port=4
  mode : Outport  Port=5
  wires:
  Deadband1/1 -> y/1  "y"
  PX4 uORB Read2/2 -> Bus Selector/1
  Bus Selector/1 -> Display2/1, <z>/1  "<z>"
  Bus Selector/2 -> Display/1, Deadband/1  "<x>"
  PX4 uORB Read2/1 -> Display4/1
  Deadband2/1 -> r/1  "r"
  Deadband/1 -> x/1  "x"
  Bus Selector/3 -> Display1/1, Deadband1/1  "<y>"
  Bus Selector/4 -> Display3/1, Deadband2/1  "<r>"
  Bus Selector/5 -> mode/1  "<mode_switch>"

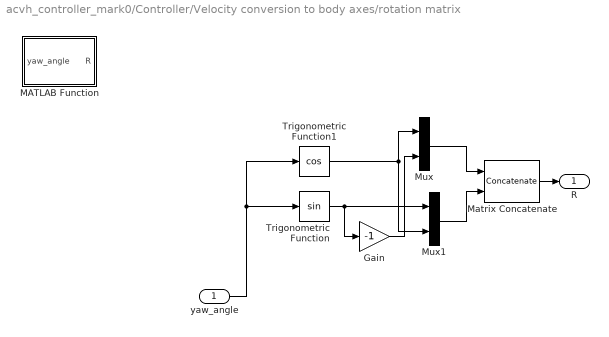
== system acvh_controller_mark0/Controller/Velocity conversion to body axes/rotation matrix ==
  yaw_angle : Inport
  Gain : Gain  Gain=-1
  MATLAB Function : MATLAB Function  TreatAsAtomicUnit=on
  Matrix Concatenate : Concatenate  Mode=Multidimensional array  ConcatenateDimension=2
  Mux : Mux  Inputs=2
  Mux1 : Mux  Inputs=2
  Trigonometric Function : Trigonometry
  Trigonometric Function1 : Trigonometry  Operator=cos
  R : Outport
  wires:
  Mux1/1 -> Matrix Concatenate/2
  Trigonometric Function1/1 -> Mux1/2, Mux/1
  yaw_angle/1 -> Trigonometric Function1/1, Trigonometric Function/1
  Trigonometric Function/1 -> Gain/1, Mux1/1
  Mux/1 -> Matrix Concatenate/1
  Gain/1 -> Mux/2
  Matrix Concatenate/1 -> R/1

== matlab function acvh_controller_mark0/Controller/Velocity conversion to body axes/rotation matrix/MATLAB Function ==
  data: yaw_angle input; R output
function R = fcn(yaw_angle)
    
R = [cos(yaw_angle) -sin(yaw_angle); sin(yaw_angle) cos(yaw_angle)];

== matlab function acvh_controller_mark0/Controller/Velocity conversion to body axes/rotation_matrix ==
  data: yaw_angle input; R output
function R = fcn(yaw_angle)
    
R = [cos(yaw_angle) -sin(yaw_angle); sin(yaw_angle) cos(yaw_angle)];
